simulink model "boost_simulink"  (R2021a)
settings: Solver=FixedStepDiscrete  StartTime=0.0  StopTime=10  FixedStep=sampleTime  MaxStep=1e-4  RelTol=1e-4  EnableMultiTasking=on
InitFcn:
  | boost_parameters
model workspace (MAT data in the model file):
  Phase1 = 0
values from neighbouring files (symbols this model uses):
  Cin = 220e-6    (= 0.00022)    [boost_parameters.m]
  D = 0.2667    [boost_parameters.m]
  Lcoil = 3.4e-3    (= 0.0034)    [boost_parameters.m]
  Lin = 1e-6    (= 1e-06)    [boost_parameters.m]
  Module1Phase = 0    [boost_parameters.m]
  Rcoil = 1e-3    (= 0.001)    [boost_parameters.m]
  Rin = 1e-3    (= 0.001)    [boost_parameters.m]
  sampleTime = 5e-7    (= 5e-07)    [boost_parameters.m]
  Vin = 880    [boost_parameters.m]
libraries: spsSeriesRLCBranchLib x6, spsMosfetLib x2, simulink x2, spsCurrentMeasurementLib x1, spsTriangleGeneratorLib x1, spsDCVoltageSourceLib x1, spsVoltageMeasurementLib x1, spspowerguiLib x1
settings Model: Creator=The MathWorks, Inc.  LastModifiedBy=enes_
settings SolverCC: AlgebraicLoopSolver=TrustRegion  SolverResetMethod=Robust
settings OptimizationCC: EfficientFloat2IntCast=on  LifeSpan=inf
settings DebuggingCC: ReadBeforeWriteMsg=DisableAll  WriteAfterWriteMsg=DisableAll  WriteAfterReadMsg=DisableAll  UniqueDataStoreMsg=error  StrictBusMsg=ErrorOnBusTreatedAsVector  SFUnexpectedBacktrackingDiag=warning  SFNoUnconditionalDefaultTransitionDiag=warning  SFExecutionAtInitializationDiag=none  SFMachineParentedDataDiag=warning  ArithmeticOperatorsInVariantConditions=warning
settings ModelReferenceCC: UpdateModelReferenceTargets=IfOutOfDate
settings SFSimCC: SFSimEcho=off  SimUseLocalCustomCode=off  CustomCodeUndefinedFunction=UseInterfaceOnly
settings RTWCC: RTWUseLocalCustomCode=off
settings CodeAppCC: StateflowObjectComments=on
settings GRTTargetCC: TargetLangStandard=C89/C90 (ANSI)
settings ConfigComp: CovMetricSettings=dw  CovSaveCumulativeToWorkspaceVar=on  CovSaveSingleToWorkspaceVar=on  CovExternalEMLEnable=off
settings SimscapeCC: SimscapeNormalizeSystem=off  SimscapeNominalValues={1, 'bar'; 1, 'cm^3/s'; 1, 'bar*kg/s'; 1, 'kJ/kg'; 1, 'kW'; }

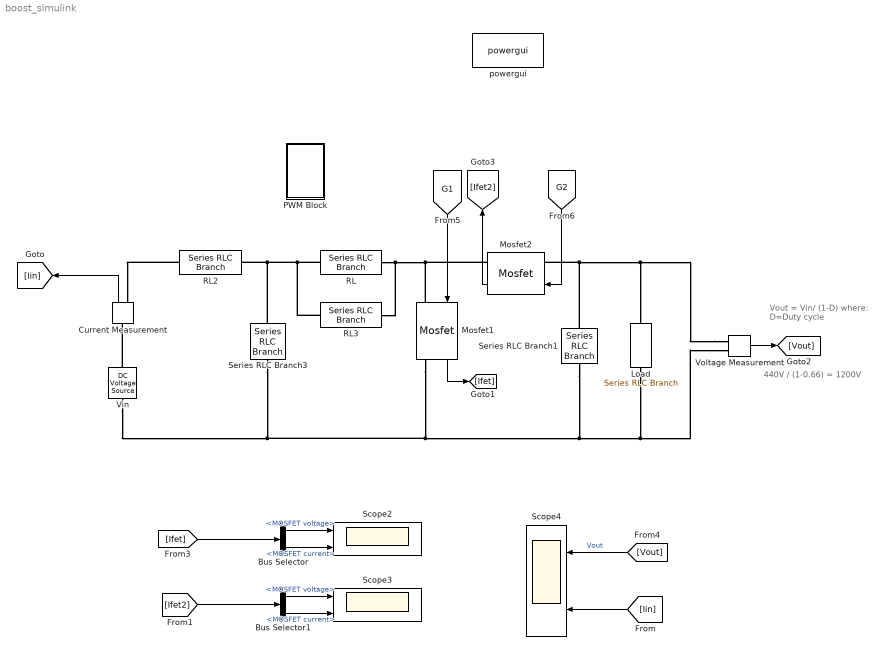
== system boost_simulink ==
  note: 440V / (1-0.66) = 1200V
  note: Vout = Vin/ (1-D)
      | where: D=Duty cycle
  Bus Selector : BusSelector  OutputSignals=MOSFET voltage,MOSFET current
  Bus Selector1 : BusSelector  OutputSignals=MOSFET voltage,MOSFET current
  Current Measurement : spsCurrentMeasurementLib/Current Measurement  PhasorSimulation=off  OutputType=Complex  PSBequivalent=0
  Load : spsSeriesRLCBranchLib/Series RLC Branch  LConnTagsString=__new0  RConnTagsString=__new0  BranchType=R  Resistance=72  Inductance=200e-6  SetiL0=off  InitialCurrent=0  Capacitance=400e-6  Setx0=off  InitialVoltage=0  Measurements=None
  Mosfet1 : spsMosfetLib/Mosfet  Ron=1e-3  Lon=0  Rd=1e-3  Vfd=0  IC=0  Rs=inf  Cs=inf  Measurements=on
  Mosfet2 : spsMosfetLib/Mosfet  Ron=1e-3  Lon=0  Rd=1e-3  Vfd=0  IC=0  Rs=inf  Cs=inf  Measurements=on
  PWM Block : Subsystem
  RL : spsSeriesRLCBranchLib/Series RLC Branch  LConnTagsString=__new0  RConnTagsString=__new0  BranchType=RL  Resistance=Rcoil  Inductance=Lcoil  SetiL0=off  InitialCurrent=8  Capacitance=1e-6  Setx0=off  InitialVoltage=0  Measurements=None
  RL2 : spsSeriesRLCBranchLib/Series RLC Branch  LConnTagsString=__new0  RConnTagsString=__new0  BranchType=RL  Resistance=Rin  Inductance=Lin  SetiL0=off  InitialCurrent=8  Capacitance=1e-6  Setx0=off  InitialVoltage=0  Measurements=None
  RL3 : spsSeriesRLCBranchLib/Series RLC Branch  LConnTagsString=__new0  RConnTagsString=__new0  BranchType=R  Resistance=1e6  Inductance=3.4e-3  SetiL0=off  InitialCurrent=8  Capacitance=1e-6  Setx0=off  InitialVoltage=0  Measurements=None
  Scope2 : Scope  NumInputPorts=2
  Scope3 : Scope  NumInputPorts=2
  Scope4 : Scope  NumInputPorts=2
  Series RLC Branch1 : spsSeriesRLCBranchLib/Series RLC Branch  LConnTagsString=__new0  RConnTagsString=__new0  BranchType=C  Resistance=1e-4  Inductance=200e-6  SetiL0=off  InitialCurrent=0  Capacitance=200e-3  Setx0=off  InitialVoltage=1200  Measurements=None
  Series RLC Branch3 : spsSeriesRLCBranchLib/Series RLC Branch  LConnTagsString=__new0  RConnTagsString=__new0  BranchType=C  Resistance=1e-4  Inductance=200e-6  SetiL0=off  InitialCurrent=0  Capacitance=Cin  Setx0=off  InitialVoltage=440  Measurements=None
  "Vin " : spsDCVoltageSourceLib/DC Voltage Source  Amplitude=Vin  Measurements=None
  Voltage Measurement : spsVoltageMeasurementLib/Voltage Measurement  PhasorSimulation=off  OutputType=Complex  PSBequivalent=0
  powergui : spspowerguiLib/powergui  Priority=1  SimulationMode=Discrete  SampleTime=sampleTime  frequency=60  Iterations=50  frequencyindice=0  Pbase=100e6  ErrMax=1e-4  UnitsV=kV  UnitsW=MW  buscounter=0  FunctionMessages=off  echomessages=off  EnableUseOfTLC=off  CurrentSourceSwitches=off  DisableSnubberDevices=off  DisableRonSwitches=off  DisableVfSwitches=off  DisplayEquations=off  AutomaticDiscreteSolvers=off  SolverType=Tustin/Backward Euler (TBE)  Interpol=off  ExternalGateDelay=off  methode=off  Ts=100  x0status=blocks  SPID=on  SwTol=0  HookPort=off  NonlinearTolerance=1e-4  nMaxIteration=100  ContinueOnMaxIteration=off  RestoreLinks=warning  ResistiveCurrentMeasurement=off  Frange=[0:2:500]  Ylog=off  Xlog=on  ShowGrid=off  save=off  variable=ZData  structure=0  ZoomFFT=off  StartTime=0.0  cycles=1  DisplayStyle=1  fundamental=60  FreqAxis=off  MaxFrequency=1000  frequencyindicesteady=1  RmsSteady=1  display=off
  wires:
  Voltage Measurement/1 -> [Vout]
  Mosfet1/1 -> [Ifet]
  Mosfet2/1 -> [Ifet2]
  Current Measurement/1 -> [Iin]
  [Ifet] -> Bus Selector/1
  Bus Selector/1 -> Scope2/1  "<MOSFET voltage>"
  Bus Selector/2 -> Scope2/2  "<MOSFET current>"
  [Vout] -> Scope4/1  "Vout"
  [G1] -> Mosfet1/1
  [G2] -> Mosfet2/1
  [Iin] -> Scope4/2
  Bus Selector1/1 -> Scope3/1  "<MOSFET voltage>"
  Bus Selector1/2 -> Scope3/2  "<MOSFET current>"
  [Ifet2] -> Bus Selector1/1
  connections:
  RL/RConn1 -- RL3/RConn1 -- Mosfet2/RConn1 -- Mosfet1/LConn1
  RL/LConn1 -- RL3/LConn1 -- Series RLC Branch3/LConn1 -- RL2/RConn1
  "Vin "/RConn1 -- Current Measurement/LConn1
  RL2/LConn1 -- Current Measurement/RConn1
  Voltage Measurement/LConn1 -- Load/LConn1 -- Series RLC Branch1/LConn1 -- Mosfet2/LConn1
  Mosfet1/RConn1 -- Series RLC Branch3/RConn1 -- "Vin "/LConn1 -- Series RLC Branch1/RConn1 -- Load/RConn1 -- Voltage Measurement/LConn2

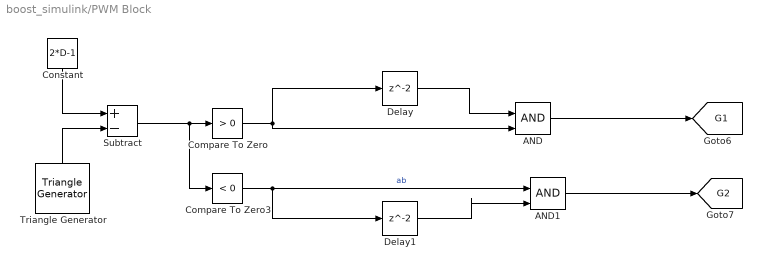
== system boost_simulink/PWM Block ==
  AND : Logic  IconShape=distinctive  AllPortsSameDT=off  OutDataTypeStr=boolean
  AND1 : Logic  IconShape=distinctive  AllPortsSameDT=off  OutDataTypeStr=boolean
  Compare To Zero : simulink/Logic and Bit Operations/Compare To Zero  relop=>  OutDataTypeStr=boolean
  Compare To Zero3 : simulink/Logic and Bit Operations/Compare To Zero  relop=<  OutDataTypeStr=boolean
  Constant : Constant  Value=2*D-1
  Delay : Delay
  Delay1 : Delay
  Subtract : Sum  Inputs=+-
  Triangle Generator : spsTriangleGeneratorLib/Triangle Generator  Freq=fsw  Phase=Module1Phase  Ts=sampleTime
  tag scope: G1=global, G2=global
  wires:
  Constant/1 -> Subtract/1
  Triangle Generator/1 -> Subtract/2
  Subtract/1 -> Compare To Zero3/1, Compare To Zero/1
  AND/1 -> [G1]
  Compare To Zero/1 -> Delay/1, AND/2
  Delay/1 -> AND/1
  Compare To Zero3/1 -> Delay1/1, AND1/1  "ab"
  AND1/1 -> [G2]
  Delay1/1 -> AND1/2
